simulink model "ASK8_Modulation"  (R2021a)
settings: Solver=VariableStepAuto  StartTime=0.0  StopTime=1e-4  MaxStep=1e-7  RelTol=1e-3
undefined symbols (not defined in the file): f_sample, Fs, gain_dB, ip, seed, usb
libraries: plutoradiolib x1, commrandsrc3 x1
settings Model: Creator=Gjorgi  LastModifiedBy=Gjorgi Vitanov

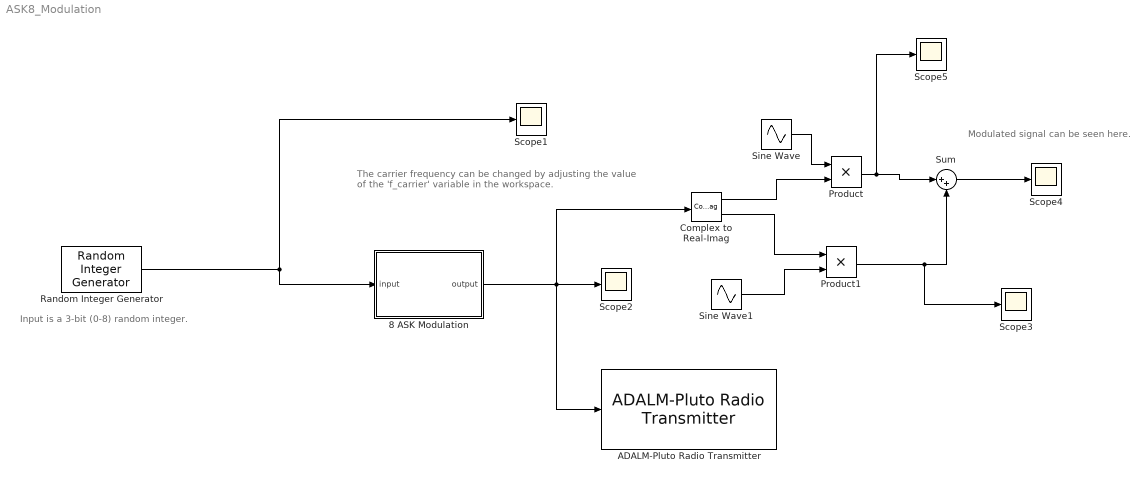
== system ASK8_Modulation ==
  note: Input is a 3-bit (0-8) random integer.
  note: The carrier frequency can be changed by adjusting the value of the 'f_carrier' variable in the workspace.
  note: Modulated signal can be seen here.
  8 ASK Modulation : MATLAB Function  TreatAsAtomicUnit=on
  ADALM-Pluto Radio Transmitter : plutoradiolib/ADALM-Pluto Radio Transmitter  RadioID=usb:0  uri=ip:10.0.0.200  CenterFrequencySource=Dialog  CenterFrequency=f_carrier  GainSource=Dialog  Gain=gain_dB  ChannelMapping=1  BasebandSampleRate=f_sample  UnderflowOutputPort=on  ShowAdvancedProperties=off  UseCustomFilter=off  filtPathRates=[737280000 11520000 3840000 1920000 960000 240000]  filtCoefficients=[-192 82 85 -215 228 -102 -110 290 -318 145 160 -426 471 -215 -238 633 -697 318 349 -923 1009 -457 -498 1309 -1423 640 693 -1812 1959 -876 -945 2458 -2647 1180 1268 -3290 3534 -1572 -1688 4375 -4698 2091 2247 -5836 6284 -2807 -3031 7918 -8588 3870 4225 -11182 12324 -5662 -6330 17255 -19735 9507 11312 -33568 43355 -25227 -42139 305542 305542 -42139 -25227 43355 -33568 11312 9507 -19735 17255 -6330 -5662 12324 -11182 4225 3870 -8588 7918 -3031 -2807 6284 -5836 2247 2091 -4698 4375 -1688 -1572 3534 -3290 1268 1180 -2647 2458 -945 -876 1959 -1812 693 640 -1423 1309 -498 -457 1009 -923 349 318 -697 633 -238 -215 471 -426 160 145 -318 290 -110 -102 228 -215 85 82 -192]  filtCoefficientSize=128  filtDecimInterpFactor=4  filtGain=-12  filtRFBandwidth=18000000  filterConfigStruct=struct()  DataSourceSelect=Input Port  DDSTone1Freq=5e3  DDSTone2Freq=10e3  DDSTone1Scale=0.5  DDSTone2Scale=0.25  DataTimeout=Inf  FrequencyCorrection=0  ENSMPinControlMode=None  BISTLoopbackMode=Disabled  BISTToneInject=Disabled  BISTSignalGen=PRBS  BISTToneFreq=Fs/32  BISTToneLevel=0
      settings: SourceProductBaseCode=PLUTO
  Complex to Real-Imag : ComplexToRealImag
  Product : Product
  Product1 : Product
  Random Integer Generator : commrandsrc3/Random Integer Generator  SetSize=8  SeedSource=Parameter  Seed=seed  SampleTime=1/f_sample  SamplesPerFrame=1  OutputDataType=double  SimulateUsing=Interpreted execution
  Scope{1..5} (5 alike) : Scope
  Sine Wave : Sin  Frequency=2*pi*f_sample  SampleTime=0
  Sine Wave1 : Sin  Frequency=2*pi*f_sample  Phase=pi/2  SampleTime=0
  Sum : Sum  Inputs=|++
  wires:
  Random Integer Generator/1 -> Scope1/1, 8 ASK Modulation/1(input)
  Sine Wave/1 -> Product/1
  Product1/1 -> Scope3/1, Sum/2
  Sine Wave1/1 -> Product1/2
  Product/1 -> Scope5/1, Sum/1
  Complex to Real-Imag/2 -> Product1/1
  Sum/1 -> Scope4/1
  8 ASK Modulation/1(output) -> ADALM-Pluto Radio Transmitter/1, Complex to Real-Imag/1, Scope2/1
  Complex to Real-Imag/1 -> Product/2

== matlab function ASK8_Modulation/8 ASK Modulation ==
  data: input input; output output
function output = fcn(input)

output = 0.125*(input + 1) + 1j*0;
